simulink model "DiskretniPID"  (R2018a)
settings: Solver=VariableStepAuto  StartTime=0.0  StopTime=500  RelTol=1e-3
values from neighbouring files (symbols this model uses):
  a = c/(pi*(h1^(3/2))*(2*R-h1))    [konstanteLinearizacija.m]
  b = 2/(pi*h1*(2*R-h1))    (= 0.663145596216)    [konstanteLinearizacija.m]
  T = 1    [konstanteLinearizacija.m]
settings Model: Creator=Asus  LastModifiedBy=Nedeljko

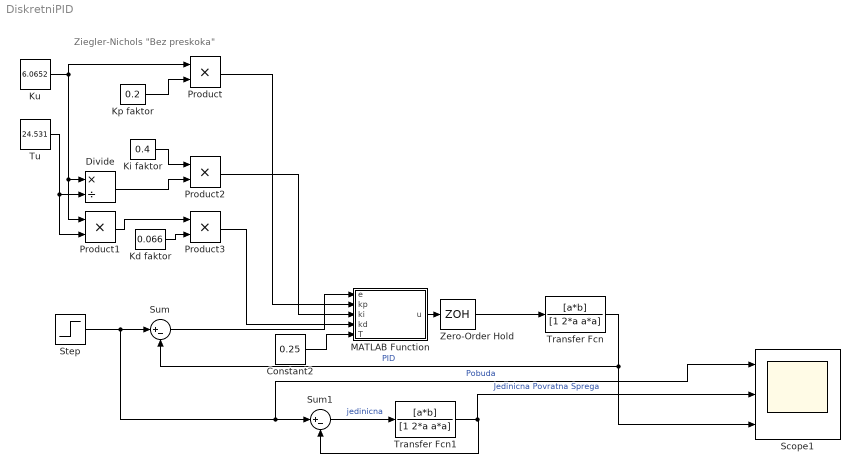
== system DiskretniPID ==
  note: Ziegler-Nichols "Bez preskoka"
  Constant2 : Constant  Value=0.25
  Divide : Product  Inputs=*/
  Kd faktor : Constant  Value=0.066
  Ki faktor : Constant  Value=0.4
  Kp faktor : Constant  Value=0.2
  Ku : Constant  Value=6.0652
  MATLAB Function : MATLAB Function  TreatAsAtomicUnit=on
  Product{,1..3} (4 alike) : Product
  Scope1 : Scope  NumInputPorts=3
  Step : Step  SampleTime=0
  Sum : Sum  Inputs=|+-
  Sum1 : Sum  Inputs=|+-
  Transfer Fcn : TransferFcn  Numerator=[a*b]  Denominator=[1 2*a a*a]
  Transfer Fcn1 : TransferFcn  Numerator=[a*b]  Denominator=[1 2*a a*a]
  Tu : Constant  Value=24.531
  Zero-Order Hold : ZeroOrderHold  SampleTime=T
  wires:
  Transfer Fcn/1 -> Sum/2, Scope1/3  "PID"
  Sum/1 -> MATLAB Function/1(e)
  Step/1 -> Scope1/1, Sum1/1, Sum/1  "Pobuda"
  Constant2/1 -> MATLAB Function/5(T)
  MATLAB Function/1(u) -> Zero-Order Hold/1
  Zero-Order Hold/1 -> Transfer Fcn/1
  Sum1/1 -> Transfer Fcn1/1  "jedinicna"
  Transfer Fcn1/1 -> Scope1/2, Sum1/2  "Jedinicna Povratna Sprega"
  Ku/1 -> Product1/1, Divide/1, Product/1
  Tu/1 -> Product1/2, Divide/2
  Kp faktor/1 -> Product/2
  Product1/1 -> Product3/1
  Divide/1 -> Product2/2
  Ki faktor/1 -> Product2/1
  Kd faktor/1 -> Product3/2
  Product/1 -> MATLAB Function/2(kp)
  Product2/1 -> MATLAB Function/3(ki)
  Product3/1 -> MATLAB Function/4(kd)

== matlab function DiskretniPID/MATLAB Function ==
  settings: updateMethod=DISCRETE
  data: e input; u output; kp input; ki input; kd input; T input
function u = fcn(e,kp,ki,kd,T)
persistent u1 e1 e2;


%inicijalizacija globalnih promenljivih
if isempty(e1)
    e1=0;
end

if isempty(e2)
    e2=0;
end

if isempty(u1)
    u1=0;
end

%upravljacki algoritam
u = u1 + e*(kp*T + ki*T^2 + kd)/T + e1*(-kp*T -2*kd)/T + e2*kd/T;

%azuriranje globalnih promenljivih
u1=u;
e2 = e1;
e1 = e;
end
